simulink library "AswLib"  (R2023b)
settings: Solver=VariableStepAuto  StartTime=0.0  StopTime=10.0  RelTol=1e-3
settings Model: Creator=84339  LastModifiedBy=84339

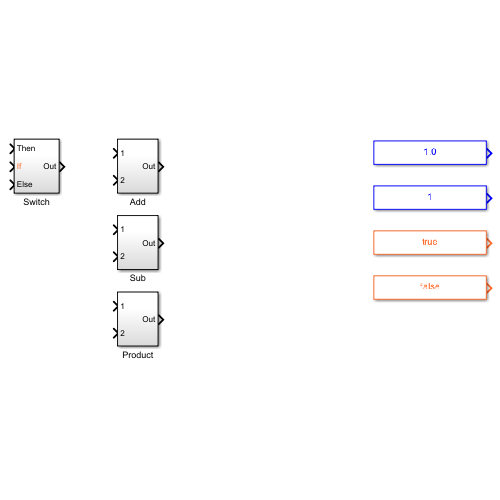
[thumbnail: Simulink's stored preview of the top-level diagram]
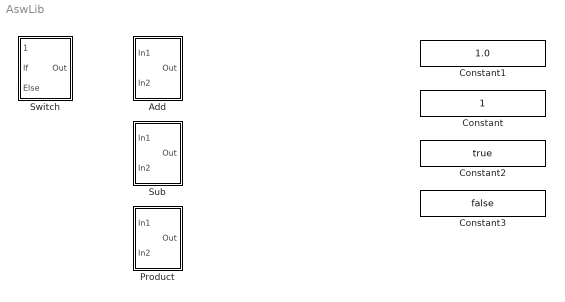
== system AswLib ==
  Add : Subsystem
  Constant : Constant
  Constant1 : Constant  Value=1.0  OutDataTypeStr=single
  Constant2 : Constant  Value=true  OutDataTypeStr=boolean
  Constant3 : Constant  Value=false  OutDataTypeStr=boolean
  Product : Subsystem
  Sub : Subsystem
  Switch : Subsystem

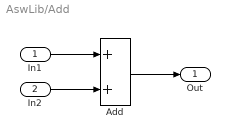
== system AswLib/Add ==
  In1 : Inport
  In2 : Inport  Port=2
  Add : Sum
  Out : Outport
  wires:
  In1/1 -> Add/1
  In2/1 -> Add/2
  Add/1 -> Out/1

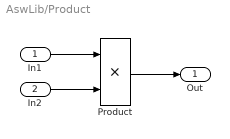
== system AswLib/Product ==
  In1 : Inport
  In2 : Inport  Port=2
  Product : Product
  Out : Outport
  wires:
  In1/1 -> Product/1
  In2/1 -> Product/2
  Product/1 -> Out/1

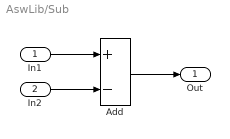
== system AswLib/Sub ==
  In1 : Inport
  In2 : Inport  Port=2
  Add : Sum  Inputs=+-
  Out : Outport
  wires:
  In1/1 -> Add/1
  In2/1 -> Add/2
  Add/1 -> Out/1

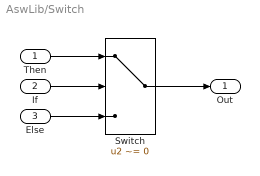
== system AswLib/Switch ==
  Then : Inport
  If : Inport  Port=2
  Else : Inport  Port=3
  Switch : Switch  Criteria=u2 ~= 0  SaturateOnIntegerOverflow=off  InputSameDT=off
  Out : Outport
  wires:
  Then/1 -> Switch/1
  Switch/1 -> Out/1
  If/1 -> Switch/2
  Else/1 -> Switch/3
